simulink model "Dual_Parallel_IPMSM_Rotate_HFI"  (R2022b)
settings: Solver=FixedStepAuto  StartTime=0.0  StopTime=20  FixedStep=1e-7  RelTol=1e-3
undefined symbols (not defined in the file): DiscIntNeverNeededParam
libraries: dsparch4 x6, slpidlib x4, spsSecondOrderFilterLib x2, spsPermanentMagnetSynchronousMachineLib x2, spsDCVoltageSourceLib x1, simulink x1, spsUniversalBridgeLib x1, spspowerguiLib x1
settings Model: Creator=SSC  LastModifiedBy=SSC

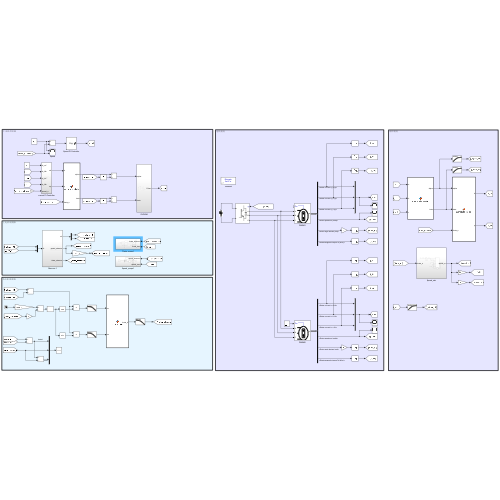
[thumbnail: Simulink's stored preview of the top-level diagram]
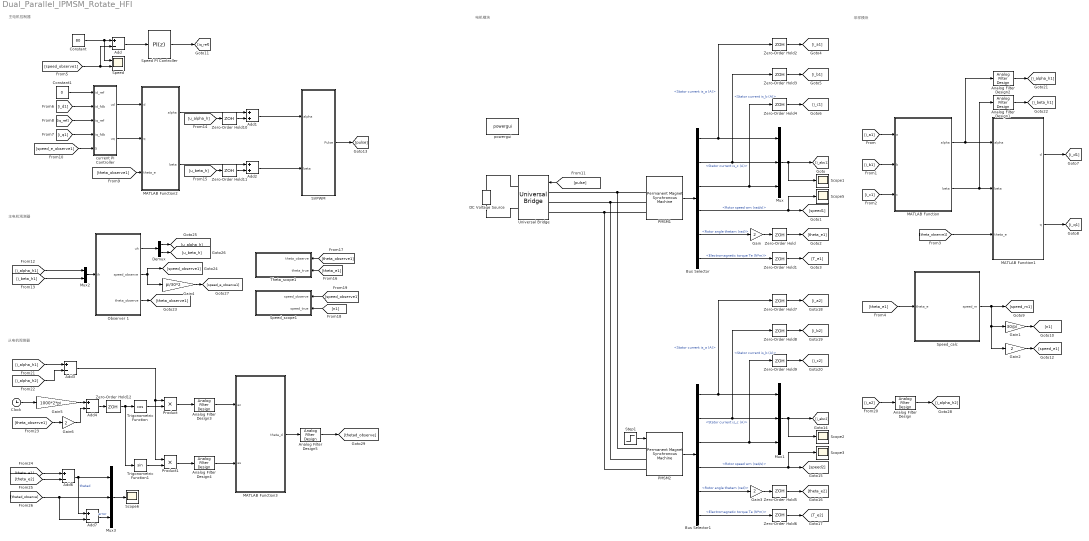
== system Dual_Parallel_IPMSM_Rotate_HFI ==
  note: 主电机观测器
  note: 采样模块
  note: 电机模块
  note: 主电机控制器
  note: 从电机观测器
  Add{,3..4,6..7} (5 alike) : Sum  Inputs=+-
  Add1 : Sum
  Add2 : Sum
  Analog Filter Design : dsparch4/Analog Filter Design  method=Butterworth  filttype=Highpass  N=1  Wlo=200*2*pi  Whi=80  Rp=2  Rs=40
  Analog Filter Design1 : dsparch4/Analog Filter Design  method=Butterworth  filttype=Highpass  N=1  Wlo=200*2*pi  Whi=80  Rp=2  Rs=40
  Analog Filter Design2 : dsparch4/Analog Filter Design  method=Butterworth  filttype=Highpass  N=1  Wlo=200*2*pi  Whi=80  Rp=2  Rs=40
  Analog Filter Design3 : dsparch4/Analog Filter Design  method=Butterworth  filttype=Lowpass  N=1  Wlo=2*2*pi  Whi=80  Rp=2  Rs=40
  Analog Filter Design4 : dsparch4/Analog Filter Design  method=Butterworth  filttype=Lowpass  N=1  Wlo=2*2*pi  Whi=80  Rp=2  Rs=40
  Analog Filter Design5 : dsparch4/Analog Filter Design  method=Butterworth  filttype=Lowpass  N=1  Wlo=1*2*pi  Whi=80  Rp=2  Rs=40
  Bus Selector : BusSelector  OutputSignals=Stator current is_a (A),Stator current is_b (A),Stator current is_c (A),Rotor speed wm (rad/s),Rotor angle thetam (rad),Electromagnetic torque Te (N*m)
  Bus Selector1 : BusSelector  OutputSignals=Stator current is_a (A),Stator current is_b (A),Stator current is_c (A),Rotor speed wm (rad/s),Rotor angle thetam (rad),Electromagnetic torque Te (N*m)
  Clock : Clock
  Constant : Constant  Value=80
  Constant1 : Constant  Value=0
  DC Voltage Source : spsDCVoltageSourceLib/DC Voltage Source  Amplitude=600  Measurements=None
  Demux : Demux  Outputs=2
  Gain{,2..3,6} (4 alike) : Gain  Gain=2
  Gain1 : Gain  Gain=30/pi
  Gain4 : Gain  Gain=pi/30*2
  Gain5 : Gain  Gain=1000*2*pi
  MATLAB Function : MATLAB Function  TreatAsAtomicUnit=on
  MATLAB Function1 : MATLAB Function  TreatAsAtomicUnit=on
  MATLAB Function2 : MATLAB Function  TreatAsAtomicUnit=on
  MATLAB Function3 : MATLAB Function  TreatAsAtomicUnit=on
  Mux : Mux  Inputs=3
  Mux1 : Mux  Inputs=3
  Mux2 : Mux  Inputs=2
  Mux3 : Mux  Inputs=3
  Observer 1 : Subsystem
  PMSM1 : spsPermanentMagnetSynchronousMachineLib/Permanent Magnet Synchronous Machine  NbPhases=3  FluxDistribution=Sinusoidal  RotorType=Salient-pole  MechanicalLoad=Torque Tm  PresetModel=No  ShowDetailedParameters=on  MeasurementBus=off  Resistance=0.91  Inductance=8.5e-3  dqInductances=[0.00396,0.00796]  La=8.5e-3  MachineConstant=Flux linkage established by magnets (V.s)  Flux=0.446  VoltageCst=161.7909  TorqueCst=1.338  Flat=120  Mechanical=[0.074 0.008 2 0]  PolePairs=4  InitialConditions=[0, 0, 0 ,0]  InitialConditions5ph=[0 0 0 0 0 0]  RefAngle=Aligned with phase A axis (original Park)  IterativeDiscreteModel=Trapezoidal non iterative  TsBlock=-1  TsPowergui=0
  PMSM2 : spsPermanentMagnetSynchronousMachineLib/Permanent Magnet Synchronous Machine  NbPhases=3  FluxDistribution=Sinusoidal  RotorType=Salient-pole  MechanicalLoad=Torque Tm  PresetModel=No  ShowDetailedParameters=on  MeasurementBus=off  Resistance=0.91  Inductance=8.5e-3  dqInductances=[0.00396,0.00796]  La=8.5e-3  MachineConstant=Flux linkage established by magnets (V.s)  Flux=0.446  VoltageCst=161.7909  TorqueCst=1.338  Flat=120  Mechanical=[0.074 0.008 2 0]  PolePairs=4  InitialConditions=[0, 0, 0 ,0]  InitialConditions5ph=[0 0 0 0 0 0]  RefAngle=Aligned with phase A axis (original Park)  IterativeDiscreteModel=Trapezoidal non iterative  TsBlock=-1  TsPowergui=0
  Product : Product
  Product1 : Product
  SVPWM : Subsystem
  Scope{1..3,5..6} (5 alike) : Scope
  Speed : Scope  NumInputPorts=2
  Speed PI Controller : slpidlib/PID Controller  Controller=PI  Form=Parallel  TimeDomain=Discrete-time  UseExternalTs=off  SampleTime=1e-4  IntegratorMethod=Forward Euler  FilterMethod=Forward Euler  ControllerParametersSource=internal  P=3.736/60  I=44.84/60  UseKiTs=off  D=0  N=100  UseFilter=on  TunerSelectOption=Transfer Function Based (PID Tuner App)  InitialConditionSource=internal  InitialConditionForIntegrator=0  InitialConditionForFilter=0  DifferentiatorICPrevScaledInput=0  ExternalReset=none  TrackingMode=off  Kt=1  LimitOutput=on  SatLimitsSource=internal  UpperSaturationLimit=20  LowerSaturationLimit=-20  LinearizeAsGain=on  AntiWindupMode=clamping  Kb=1  LimitIntegrator=off  UpperIntegratorSaturationLimit=5.65  LowerIntegratorSaturationLimit=-inf  POutMin=[]  POutMax=[]  IOutMin=[]  IOutMax=[]  DOutMin=[]  DOutMax=[]  NOutMin=[]  NOutMax=[]  SumOutMin=[]  SumOutMax=[]  SaturationOutMin=[]  SaturationOutMax=[]  PParamMin=[]  PParamMax=[]  IParamMin=[]  IParamMax=[]  DParamMin=[]  DParamMax=[]  NParamMin=[]  NParamMax=[]  KbParamMin=[]  KbParamMax=[]  KtParamMin=[]  KtParamMax=[]  KbOutMin=[]  KbOutMax=[]  KtOutMin=[]  KtOutMax=[]  IntegratorOutMin=[]  IntegratorOutMax=[]  FilterOutMin=[]  FilterOutMax=[]  SumI1OutMin=[]  SumI1OutMax=[]  SumI2OutMin=[]  SumI2OutMax=[]  SumI3OutMin=[]  SumI3OutMax=[]  SumI4OutMin=[]  SumI4OutMax=[]  SumDOutMin=[]  SumDOutMax=[]  DifferentiatorOutMin=[]  DifferentiatorOutMax=[]  FilterDiffOutCoefMin=[]  FilterDiffOutCoefMax=[]  ReciprocalOutMin=[]  ReciprocalOutMax=[]  SumDenOutMin=[]  SumDenOutMax=[]  SumNumOutMin=[]  SumNumOutMax=[]  DivideOutMin=[]  DivideOutMax=[]  UdiffTsProdOutMin=[]  UdiffTsProdOutMax=[]  NTsProdOutMin=[]  NTsProdOutMax=[]  UintegralTsProdOutMin=[]  UintegralTsProdOutMax=[]  UngainTsProdOutMin=[]  UngainTsProdOutMax=[]  ClampingZeroOutDataTypeStr=Inherit: Inherit via back propagation  ClampingZeroOutMin=[]  ClampingZeroOutMax=[]  FilterDenConstantOutDataTypeStr=Inherit: Inherit via back propagation  FilterDenConstantOutMin=[]  FilterDenConstantOutMax=[]  PCopyOutDataTypeStr=Inherit: Inherit via back propagation  PCopyOutMin=[]  PCopyOutMax=[]  NCopyOutDataTypeStr=Inherit: Inherit via back propagation  NCopyOutMin=[]  NCopyOutMax=[]  IntegratorContinuousStateAttributes=''  IntegratorStateMustResolveToSignalObject=off  IntegratorRTWStateStorageClass=Auto  FilterContinuousStateAttributes=''  FilterStateMustResolveToSignalObject=off  FilterRTWStateStorageClass=Auto  ParallelPVariant=InternalParameters  IdealPVariant=Disabled  IVariant=InternalParameters  DVariant=Disabled  IntegratorVariant=Discrete  SatVariant=Enabled  AWVariant=DiscClampingParallel  PCopyVariant=Disabled  TRVariant=Disabled  FdbkBlocksVariant=Forward  IdealPFdbkVariant=Disabled  SatFdbkVariant=Disabled  DerivativeFilterVariant=Disabled  NVariant=Disabled  NCopyVariant=Disabled_SignalSpec  FilterICVariant=Disabled  IntegratorICVariant=InternalICs  ExternalResetVariant=Disabled  TRSumVariant=Passthrough  SumFdbkVariant=Disabled  SumVariant=Sum_PI  TsampFilterVariant=InternalTs  TsampNgainVariant=Passthrough  TsampIntegralVariant=Passthrough  ExternalSaturationOutDataTypeStr=Inherit: Same as second input
  Speed_calc : Subsystem
  Speed_scope1 : Subsystem
  Step1 : Step  After=0.01  SampleTime=0
  Theta_scope1 : Subsystem
  Trigonometric Function : Trigonometry  Operator=cos
  Trigonometric Function1 : Trigonometry
  Universal Bridge : spsUniversalBridgeLib/Universal Bridge  Arms=3  SnubberResistance=1e5  SnubberCapacitance=inf  Device=IGBT / Diodes  Ron=1e-3  Lon=0  ForwardVoltages="[  0  0  ]"  ForwardVoltage=0  GTOparameters=[ 10e-6 , 20e-6 ]  IGBTparameters=[ 1e-6 , 2e-6 ]  Measurements=None  Measurements_2=None  converterType=Rectifier
  Zero-Order Hold{,1..12} (13 alike) : ZeroOrderHold  SampleTime=1e-4
  current PI Controller : Subsystem
  powergui : spspowerguiLib/powergui  Priority=1  SimulationMode=Discrete  SampleTime=5e-7  frequency=60  Iterations=50  frequencyindice=0  Pbase=100e6  ErrMax=1e-4  UnitsV=kV  UnitsW=MW  buscounter=0  FunctionMessages=off  echomessages=off  EnableUseOfTLC=off  CurrentSourceSwitches=off  DisableSnubberDevices=off  DisableRonSwitches=off  DisableVfSwitches=off  DisplayEquations=off  AutomaticDiscreteSolvers=off  SolverType=Tustin/Backward Euler (TBE)  Interpol=off  ExternalGateDelay=off  methode=off  Ts=100  x0status=blocks  SPID=on  SwTol=0  HookPort=off  NonlinearTolerance=1e-4  nMaxIteration=100  ContinueOnMaxIteration=off  RestoreLinks=warning  ResistiveCurrentMeasurement=off  Frange=[0:2:500]  Ylog=off  Xlog=on  ShowGrid=off  save=off  variable=ZData  structure=0  ZoomFFT=off  StartTime=0.0  cycles=1  DisplayStyle=1  fundamental=60  FreqAxis=off  MaxFrequency=1000  frequencyindicesteady=1  RmsSteady=1  display=off
  wires:
  Zero-Order Hold4/1 -> [i_c1]
  current PI Controller/2(uq) -> MATLAB Function2/2(q)
  Constant1/1 -> current PI Controller/1(id_ref)
  [theta_observe1] -> MATLAB Function1/3(theta_e)
  SVPWM/1(Pulse) -> [pulse]
  current PI Controller/1(ud) -> MATLAB Function2/1(d)
  Speed PI Controller/1 -> [iq_ref]
  [theta_observe1] -> MATLAB Function2/3(theta_e)
  [iq_ref] -> current PI Controller/3(iq_ref)
  [speed_e_observe1] -> current PI Controller/5(speed_e)
  Speed_calc/1(speed_m) -> Gain2/1, Gain1/1, [speed_m1]
  Constant/1 -> Speed/1, Add/1
  Bus Selector/6 -> Zero-Order Hold1/1  "<Electromagnetic torque Te (N*m)>"
  Gain2/1 -> [speed_e1]
  PMSM1/1 -> Bus Selector/1
  MATLAB Function1/1(d) -> [i_d1]
  Add/1 -> Speed PI Controller/1
  [i_b1] -> MATLAB Function/2(b)
  [i_c1] -> MATLAB Function/3(c)
  Gain1/1 -> [n1]
  MATLAB Function1/2(q) -> [i_q1]
  [pulse] -> Universal Bridge/1
  Zero-Order Hold1/1 -> [T_e1]
  Bus Selector/1 -> Zero-Order Hold2/1, Mux/1  "<Stator current is_a (A)>"
  Bus Selector/5 -> Gain/1  "<Rotor angle thetam (rad)>"
  Bus Selector/2 -> Zero-Order Hold3/1, Mux/2  "<Stator current is_b (A)>"
  Mux/1 -> Scope1/1, [i_abc1]
  Gain/1 -> Zero-Order Hold/1
  Bus Selector/3 -> Zero-Order Hold4/1, Mux/3  "<Stator current is_c (A)>"
  [speed_observe1] -> Add/2, Speed/2
  Zero-Order Hold2/1 -> [i_a1]
  Zero-Order Hold/1 -> [theta_e1]
  [i_d1] -> current PI Controller/2(id_fdb)
  MATLAB Function/2(beta) -> Analog Filter Design1/1, MATLAB Function1/2(beta)
  [theta_e1] -> Speed_calc/1(theta_e)
  Zero-Order Hold3/1 -> [i_b1]
  [i_a1] -> MATLAB Function/1(a)
  Bus Selector/4 -> Scope5/1, [speed1]  "<Rotor speed wm (rad/s)>"
  MATLAB Function/1(alpha) -> Analog Filter Design2/1, MATLAB Function1/1(alpha)
  [i_q1] -> current PI Controller/4(iq_fdb)
  Zero-Order Hold5/1 -> [theta_e2]
  Zero-Order Hold8/1 -> [i_b2]
  Bus Selector1/3 -> Zero-Order Hold9/1, Mux1/3  "<Stator current is_c (A)>"
  Zero-Order Hold7/1 -> [i_a2]
  Bus Selector1/1 -> Zero-Order Hold7/1, Mux1/1  "<Stator current is_a (A)>"
  Bus Selector1/4 -> Scope3/1, [speed2]  "<Rotor speed wm (rad/s)>"
  Bus Selector1/6 -> Zero-Order Hold6/1  "<Electromagnetic torque Te (N*m)>"
  Gain3/1 -> Zero-Order Hold5/1
  Bus Selector1/2 -> Zero-Order Hold8/1, Mux1/2  "<Stator current is_b (A)>"
  Zero-Order Hold6/1 -> [T_e2]
  Mux1/1 -> Scope2/1, [i_abc2]
  PMSM2/1 -> Bus Selector1/1
  Zero-Order Hold9/1 -> [i_c2]
  Bus Selector1/5 -> Gain3/1  "<Rotor angle thetam (rad)>"
  MATLAB Function2/1(alpha) -> Add1/1
  MATLAB Function2/2(beta) -> Add2/1
  Zero-Order Hold10/1 -> Add1/2
  Zero-Order Hold11/1 -> Add2/2
  Analog Filter Design1/1 -> [i_beta_h1]
  Analog Filter Design2/1 -> [i_alpha_h1]
  Observer 1/1(uh) -> Demux/1
  Mux2/1 -> Observer 1/1(ih)
  [i_alpha_h1] -> Mux2/1
  [i_beta_h1] -> Mux2/2
  Observer 1/3(theta_observe) -> [theta_observe1]
  Observer 1/2(speed_observe) -> [speed_observe1], Gain4/1
  [u_alpha_h] -> Zero-Order Hold10/1
  [u_beta_h] -> Zero-Order Hold11/1
  Demux/2 -> [u_beta_h]
  Demux/1 -> [u_alpha_h]
  [theta_observe1] -> Theta_scope1/1(theta_observe)
  [theta_e1] -> Theta_scope1/2(theta_true)
  [n1] -> Speed_scope1/2(speed_true)
  [speed_observe1] -> Speed_scope1/1(speed_observe)
  Gain4/1 -> [speed_e_observe1]
  Analog Filter Design/1 -> [i_alpha_h2]
  [i_a2] -> Analog Filter Design/1
  [i_alpha_h1] -> Add3/1
  [i_alpha_h2] -> Add3/2
  Clock/1 -> Gain5/1
  Gain5/1 -> Add4/1
  [theta_observe1] -> Gain6/1
  Add3/1 -> Product1/1, Product/1
  Product/1 -> Analog Filter Design3/1
  Trigonometric Function1/1 -> Product1/2
  Product1/1 -> Analog Filter Design4/1
  Analog Filter Design3/1 -> MATLAB Function3/1(ec)
  Analog Filter Design4/1 -> MATLAB Function3/2(es)
  [theta_e1] -> Add6/1
  [theta_e2] -> Add6/2
  Add6/1 -> Mux3/1, Add7/1  "thetad"
  [thetad_observe] -> Add7/2, Mux3/2
  Mux3/1 -> Scope6/1
  Add7/1 -> Mux3/3  "error"
  Add1/1 -> SVPWM/1(alpha)
  Add2/1 -> SVPWM/2(beta)
  Gain6/1 -> Add4/2
  Trigonometric Function/1 -> Product/2
  Add4/1 -> Zero-Order Hold12/1
  Zero-Order Hold12/1 -> Trigonometric Function1/1, Trigonometric Function/1
  MATLAB Function3/1(theta_d) -> Analog Filter Design5/1
  Analog Filter Design5/1 -> [thetad_observe]
  Step1/1 -> PMSM2/1
  connections:
  Universal Bridge/RConn1 -- DC Voltage Source/RConn1
  PMSM1/LConn2 -- PMSM2/LConn2 -- Universal Bridge/LConn2
  DC Voltage Source/LConn1 -- Universal Bridge/RConn2
  PMSM1/LConn1 -- PMSM2/LConn1 -- Universal Bridge/LConn1
  PMSM1/LConn3 -- PMSM2/LConn3 -- Universal Bridge/LConn3

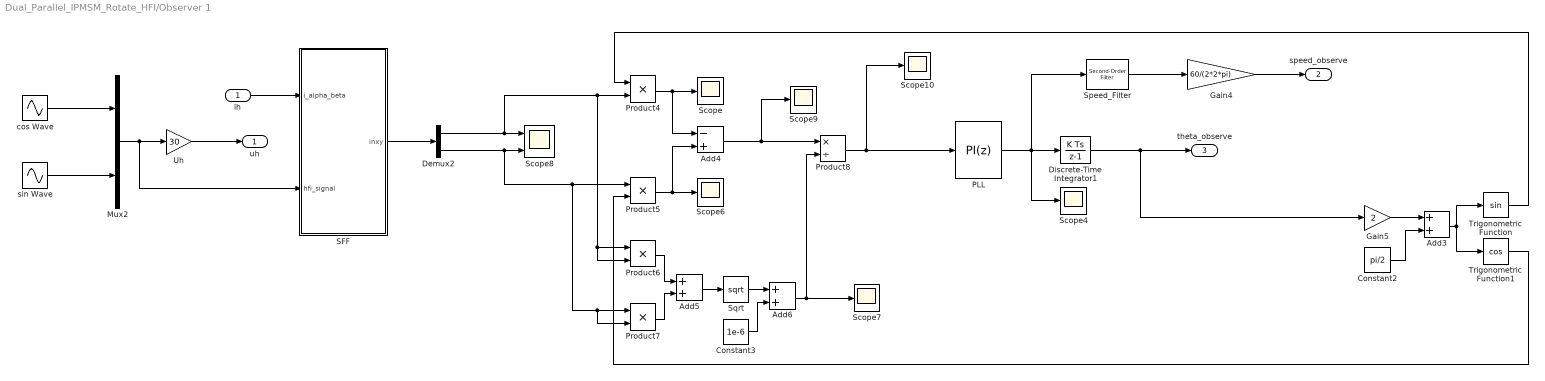
== system Dual_Parallel_IPMSM_Rotate_HFI/Observer 1 ==
  ih : Inport
  Add3 : Sum
  Add4 : Sum  Inputs=-+
  Add5 : Sum
  Add6 : Sum
  Constant2 : Constant  Value=pi/2  SampleTime=-1
  Constant3 : Constant  Value=1e-6  SampleTime=-1
  Demux2 : Demux  Outputs=2
  Discrete-Time Integrator1 : DiscreteIntegrator  SampleTime=-1  ICPrevOutput=DiscIntNeverNeededParam  ICPrevScaledInput=DiscIntNeverNeededParam
  Gain4 : Gain  Gain=60/(2*2*pi)
  Gain5 : Gain  Gain=2
  Mux2 : Mux  Inputs=2
  PLL : slpidlib/PID Controller  Controller=PI  Form=Parallel  TimeDomain=Discrete-time  UseExternalTs=off  SampleTime=1e-4  IntegratorMethod=Forward Euler  FilterMethod=Forward Euler  ControllerParametersSource=internal  P=500  I=4000  UseKiTs=off  D=0  N=100  UseFilter=on  TunerSelectOption=Transfer Function Based (PID Tuner App)  InitialConditionSource=internal  InitialConditionForIntegrator=0  InitialConditionForFilter=0  DifferentiatorICPrevScaledInput=0  ExternalReset=none  TrackingMode=off  Kt=1  LimitOutput=on  SatLimitsSource=internal  UpperSaturationLimit=100*2*pi  LowerSaturationLimit=-100*2*pi  LinearizeAsGain=on  AntiWindupMode=clamping  Kb=1  LimitIntegrator=off  UpperIntegratorSaturationLimit=inf  LowerIntegratorSaturationLimit=-inf  POutMin=[]  POutMax=[]  IOutMin=[]  IOutMax=[]  DOutMin=[]  DOutMax=[]  NOutMin=[]  NOutMax=[]  SumOutMin=[]  SumOutMax=[]  SaturationOutMin=[]  SaturationOutMax=[]  PParamMin=[]  PParamMax=[]  IParamMin=[]  IParamMax=[]  DParamMin=[]  DParamMax=[]  NParamMin=[]  NParamMax=[]  KbParamMin=[]  KbParamMax=[]  KtParamMin=[]  KtParamMax=[]  KbOutMin=[]  KbOutMax=[]  KtOutMin=[]  KtOutMax=[]  IntegratorOutMin=[]  IntegratorOutMax=[]  FilterOutMin=[]  FilterOutMax=[]  SumI1OutMin=[]  SumI1OutMax=[]  SumI2OutMin=[]  SumI2OutMax=[]  SumI3OutMin=[]  SumI3OutMax=[]  SumI4OutMin=[]  SumI4OutMax=[]  SumDOutMin=[]  SumDOutMax=[]  DifferentiatorOutMin=[]  DifferentiatorOutMax=[]  FilterDiffOutCoefMin=[]  FilterDiffOutCoefMax=[]  ReciprocalOutMin=[]  ReciprocalOutMax=[]  SumDenOutMin=[]  SumDenOutMax=[]  SumNumOutMin=[]  SumNumOutMax=[]  DivideOutMin=[]  DivideOutMax=[]  UdiffTsProdOutMin=[]  UdiffTsProdOutMax=[]  NTsProdOutMin=[]  NTsProdOutMax=[]  UintegralTsProdOutMin=[]  UintegralTsProdOutMax=[]  UngainTsProdOutMin=[]  UngainTsProdOutMax=[]  ClampingZeroOutDataTypeStr=Inherit: Inherit via back propagation  ClampingZeroOutMin=[]  ClampingZeroOutMax=[]  FilterDenConstantOutDataTypeStr=Inherit: Inherit via back propagation  FilterDenConstantOutMin=[]  FilterDenConstantOutMax=[]  PCopyOutDataTypeStr=Inherit: Inherit via back propagation  PCopyOutMin=[]  PCopyOutMax=[]  NCopyOutDataTypeStr=Inherit: Inherit via back propagation  NCopyOutMin=[]  NCopyOutMax=[]  IntegratorContinuousStateAttributes=''  IntegratorStateMustResolveToSignalObject=off  IntegratorRTWStateStorageClass=Auto  FilterContinuousStateAttributes=''  FilterStateMustResolveToSignalObject=off  FilterRTWStateStorageClass=Auto  ParallelPVariant=InternalParameters  IdealPVariant=Disabled  IVariant=InternalParameters  DVariant=Disabled  IntegratorVariant=Discrete  SatVariant=Enabled  AWVariant=DiscClampingParallel  PCopyVariant=Disabled  TRVariant=Disabled  FdbkBlocksVariant=Forward  IdealPFdbkVariant=Disabled  SatFdbkVariant=Disabled  DerivativeFilterVariant=Disabled  NVariant=Disabled  NCopyVariant=Disabled_SignalSpec  FilterICVariant=Disabled  IntegratorICVariant=InternalICs  ExternalResetVariant=Disabled  TRSumVariant=Passthrough  SumFdbkVariant=Disabled  SumVariant=Sum_PI  TsampFilterVariant=InternalTs  TsampNgainVariant=Passthrough  TsampIntegralVariant=Passthrough  ExternalSaturationOutDataTypeStr=Inherit: Same as second input
  Product{4..7} (4 alike) : Product
  Product8 : Product  Inputs=*/
  SFF : Subsystem
  Scope{,4,6..7,9..10} (6 alike) : Scope
  Scope8 : Scope  NumInputPorts=2
  Speed_Filter : spsSecondOrderFilterLib/Second-Order Filter  FilterType=Lowpass  Fo=500  Zeta=0.3  Ts=1e-4  Initialize=off  Vac_Init="[0,  0,  60]"  Vdc_Init=0  PlotResponse=off  FreqRange=[0, 500, 1]
      settings: LibrarySourceBlock=|
      | sps_lib/Control/Filters/Second-Order
      | Filter
  Sqrt : Sqrt
  Trigonometric Function : Trigonometry
  Trigonometric Function1 : Trigonometry  Operator=cos
  Uh : Gain  Gain=30
  cos Wave : Sin  Frequency=1000*2*pi  Phase=pi/2
  sin Wave : Sin  Frequency=1000*2*pi
  uh : Outport
  speed_observe : Outport  Port=2  VectorParamsAs1DForOutWhenUnconnected=off
  theta_observe : Outport  Port=3  VectorParamsAs1DForOutWhenUnconnected=off
  wires:
  Constant3/1 -> Add6/2
  ih/1 -> SFF/1(i_alpha_beta)
  Product4/1 -> Add4/1, Scope/1
  Constant2/1 -> Add3/2
  SFF/1(inxy) -> Demux2/1
  Product8/1 -> PLL/1, Scope10/1
  Sqrt/1 -> Add6/1
  Add6/1 -> Product8/2, Scope7/1
  Demux2/1 -> Product6/2, Product6/1, Product4/2, Scope8/1
  PLL/1 -> Scope4/1, Speed_Filter/1, Discrete-Time Integrator1/1
  Product5/1 -> Scope6/1, Add4/2
  cos Wave/1 -> Mux2/1
  Product7/1 -> Add5/2
  Uh/1 -> uh/1
  Add3/1 -> Trigonometric Function/1, Trigonometric Function1/1
  Add5/1 -> Sqrt/1
  Product6/1 -> Add5/1
  Gain4/1 -> speed_observe/1
  Mux2/1 -> SFF/2(hfi_signal), Uh/1
  Add4/1 -> Scope9/1, Product8/1
  Trigonometric Function/1 -> Product4/1
  Speed_Filter/1 -> Gain4/1
  Gain5/1 -> Add3/1
  Discrete-Time Integrator1/1 -> theta_observe/1, Gain5/1
  Demux2/2 -> Product7/2, Product7/1, Product5/1, Scope8/2
  sin Wave/1 -> Mux2/2
  Trigonometric Function1/1 -> Product5/2

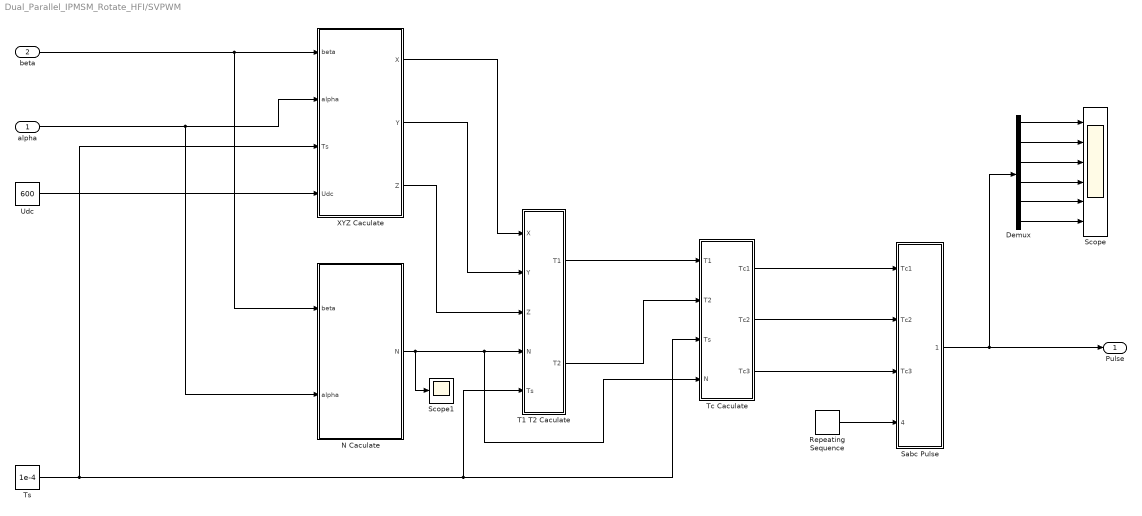
== system Dual_Parallel_IPMSM_Rotate_HFI/SVPWM ==
  alpha : Inport
  beta : Inport  Port=2
  Demux : Demux  Outputs=6
  N Caculate : Subsystem
  Repeating Sequence : simulink/Sources/Repeating Sequence  rep_seq_t=[0 0.5*1e-4 1e-4]  rep_seq_y=[0 0.5*1e-4 0]
  Sabc Pulse : Subsystem
  Scope : Scope  NumInputPorts=6
  Scope1 : Scope
  T1 T2 Caculate : Subsystem
  Tc Caculate : Subsystem
  Ts : Constant  Value=1e-4
  "Udc " : Constant  Value=600
  XYZ Caculate : Subsystem
  Pulse : Outport  VectorParamsAs1DForOutWhenUnconnected=off
  wires:
  beta/1 -> N Caculate/1(beta), XYZ Caculate/1(beta)
  alpha/1 -> N Caculate/2(alpha), XYZ Caculate/2(alpha)
  XYZ Caculate/1(X) -> T1 T2 Caculate/1(X)
  XYZ Caculate/2(Y) -> T1 T2 Caculate/2(Y)
  XYZ Caculate/3(Z) -> T1 T2 Caculate/3(Z)
  N Caculate/1(N) -> Scope1/1, Tc Caculate/4(N), T1 T2 Caculate/4(N)
  Ts/1 -> XYZ Caculate/3("Ts "), Tc Caculate/3(Ts), T1 T2 Caculate/5("Ts ")
  T1 T2 Caculate/1(T1) -> Tc Caculate/1(T1)
  T1 T2 Caculate/2(T2) -> Tc Caculate/2(T2)
  Tc Caculate/1(Tc1) -> Sabc Pulse/1(Tc1)
  Tc Caculate/2(Tc2) -> Sabc Pulse/2(Tc2)
  Tc Caculate/3(Tc3) -> Sabc Pulse/3(Tc3)
  Sabc Pulse/1("Pulse ") -> Demux/1, Pulse/1
  "Udc "/1 -> XYZ Caculate/4(Udc)
  Repeating Sequence/1 -> Sabc Pulse/4(Wave)
  Demux/1 -> Scope/1
  Demux/2 -> Scope/2
  Demux/3 -> Scope/3
  Demux/4 -> Scope/4
  Demux/5 -> Scope/5
  Demux/6 -> Scope/6

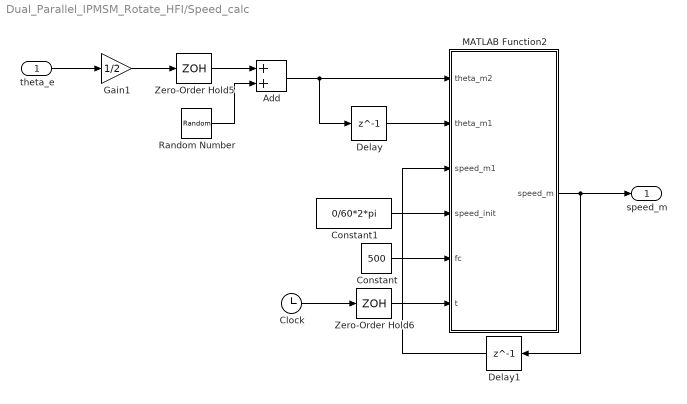
== system Dual_Parallel_IPMSM_Rotate_HFI/Speed_calc ==
  theta_e : Inport
  Add : Sum
  Clock : Clock
  Constant : Constant  Value=500
  Constant1 : Constant  Value=0/60*2*pi
  Delay : Delay  DelayLength=1  InitialCondition=0
  Delay1 : Delay  DelayLength=1  InitialCondition=0
  Gain1 : Gain  Gain=1/2
  MATLAB Function2 : MATLAB Function  TreatAsAtomicUnit=on
  Random Number : RandomNumber  Mean=1.25e-9  Variance=1.25e-9  SampleTime=1e-4
  Zero-Order Hold5 : ZeroOrderHold  SampleTime=1e-4
  Zero-Order Hold6 : ZeroOrderHold  SampleTime=1e-4
  speed_m : Outport
  wires:
  Delay/1 -> MATLAB Function2/2(theta_m1)
  Constant1/1 -> MATLAB Function2/4(speed_init)
  Clock/1 -> Zero-Order Hold6/1
  Add/1 -> Delay/1, MATLAB Function2/1(theta_m2)
  Constant/1 -> MATLAB Function2/5(fc)
  Delay1/1 -> MATLAB Function2/3(speed_m1)
  MATLAB Function2/1(speed_m) -> speed_m/1, Delay1/1
  theta_e/1 -> Gain1/1
  Zero-Order Hold6/1 -> MATLAB Function2/6(t)
  Zero-Order Hold5/1 -> Add/1
  Gain1/1 -> Zero-Order Hold5/1
  Random Number/1 -> Add/2

== system Dual_Parallel_IPMSM_Rotate_HFI/Speed_scope1 ==
  speed_observe : Inport
  speed_true : Inport  Port=2
  Add : Sum  Inputs=+-
  Mux : Mux  Inputs=3
  speed : Scope
  wires:
  Mux/1 -> speed/1
  speed_true/1 -> Mux/2, Add/1
  speed_observe/1 -> Mux/1, Add/2
  Add/1 -> Mux/3  "speed_error"

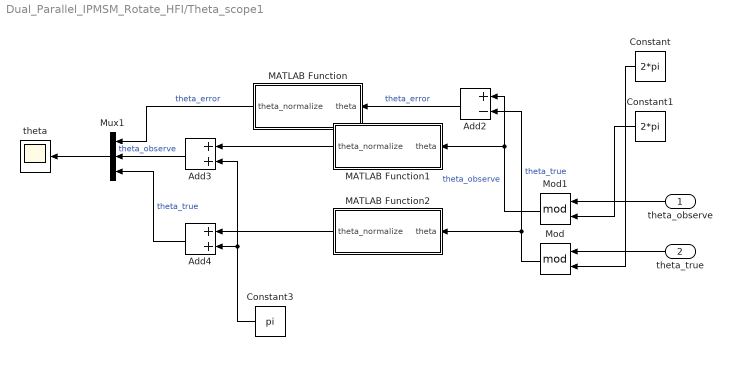
== system Dual_Parallel_IPMSM_Rotate_HFI/Theta_scope1 ==
  theta_observe : Inport
  theta_true : Inport  Port=2
  Add2 : Sum  Inputs=+-
  Add3 : Sum
  Add4 : Sum
  Constant : Constant  Value=2*pi
  Constant1 : Constant  Value=2*pi
  Constant3 : Constant  Value=pi
  MATLAB Function : MATLAB Function  TreatAsAtomicUnit=on
  MATLAB Function1 : MATLAB Function  TreatAsAtomicUnit=on
  MATLAB Function2 : MATLAB Function  TreatAsAtomicUnit=on
  Mod : Math  Operator=mod  SignedPower=on
  Mod1 : Math  Operator=mod  SignedPower=on
  Mux1 : Mux  Inputs=3
  theta : Scope
  wires:
  Add4/1 -> Mux1/3  "theta_true"
  Constant1/1 -> Mod1/2
  Constant/1 -> Mod/2
  MATLAB Function2/1(theta_normalize) -> Add4/1
  Mod/1 -> Add2/2, MATLAB Function2/1(theta)  "theta_true"
  Mux1/1 -> theta/1
  theta_observe/1 -> Mod1/1
  Constant3/1 -> Add4/2, Add3/2
  MATLAB Function/1(theta_normalize) -> Mux1/1  "theta_error"
  MATLAB Function1/1(theta_normalize) -> Add3/1
  Mod1/1 -> Add2/1, MATLAB Function1/1(theta)  "theta_observe"
  Add3/1 -> Mux1/2  "theta_observe"
  Add2/1 -> MATLAB Function/1(theta)  "theta_error"
  theta_true/1 -> Mod/1

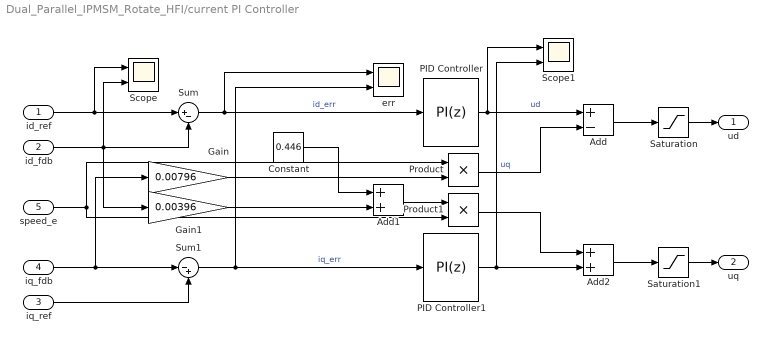
== system Dual_Parallel_IPMSM_Rotate_HFI/current PI Controller ==
  id_ref : Inport
  id_fdb : Inport  Port=2
  iq_ref : Inport  Port=3
  iq_fdb : Inport  Port=4
  speed_e : Inport  Port=5
  Add : Sum  Inputs=+-
  Add1 : Sum
  Add2 : Sum
  Constant : Constant  Value=0.446
  Gain : Gain  Gain=0.00796
  Gain1 : Gain  Gain=0.00396
  PID Controller : slpidlib/PID Controller  Controller=PI  Form=Parallel  TimeDomain=Discrete-time  UseExternalTs=off  SampleTime=1e-4  IntegratorMethod=Forward Euler  FilterMethod=Forward Euler  ControllerParametersSource=internal  P=0.00396 * 400  I=0.91 * 400  UseKiTs=off  D=0  N=100  UseFilter=on  TunerSelectOption=Transfer Function Based (PID Tuner App)  InitialConditionSource=internal  InitialConditionForIntegrator=0  InitialConditionForFilter=0  DifferentiatorICPrevScaledInput=0  ExternalReset=none  TrackingMode=off  Kt=1  LimitOutput=on  SatLimitsSource=internal  UpperSaturationLimit=600/sqrt(3)  LowerSaturationLimit=-600/sqrt(3)  LinearizeAsGain=on  AntiWindupMode=clamping  Kb=1  LimitIntegrator=off  UpperIntegratorSaturationLimit=inf  LowerIntegratorSaturationLimit=-inf  POutMin=[]  POutMax=[]  IOutMin=[]  IOutMax=[]  DOutMin=[]  DOutMax=[]  NOutMin=[]  NOutMax=[]  SumOutMin=[]  SumOutMax=[]  SaturationOutMin=[]  SaturationOutMax=[]  PParamMin=[]  PParamMax=[]  IParamMin=[]  IParamMax=[]  DParamMin=[]  DParamMax=[]  NParamMin=[]  NParamMax=[]  KbParamMin=[]  KbParamMax=[]  KtParamMin=[]  KtParamMax=[]  KbOutMin=[]  KbOutMax=[]  KtOutMin=[]  KtOutMax=[]  IntegratorOutMin=[]  IntegratorOutMax=[]  FilterOutMin=[]  FilterOutMax=[]  SumI1OutMin=[]  SumI1OutMax=[]  SumI2OutMin=[]  SumI2OutMax=[]  SumI3OutMin=[]  SumI3OutMax=[]  SumI4OutMin=[]  SumI4OutMax=[]  SumDOutMin=[]  SumDOutMax=[]  DifferentiatorOutMin=[]  DifferentiatorOutMax=[]  FilterDiffOutCoefMin=[]  FilterDiffOutCoefMax=[]  ReciprocalOutMin=[]  ReciprocalOutMax=[]  SumDenOutMin=[]  SumDenOutMax=[]  SumNumOutMin=[]  SumNumOutMax=[]  DivideOutMin=[]  DivideOutMax=[]  UdiffTsProdOutMin=[]  UdiffTsProdOutMax=[]  NTsProdOutMin=[]  NTsProdOutMax=[]  UintegralTsProdOutMin=[]  UintegralTsProdOutMax=[]  UngainTsProdOutMin=[]  UngainTsProdOutMax=[]  ClampingZeroOutDataTypeStr=Inherit: Inherit via back propagation  ClampingZeroOutMin=[]  ClampingZeroOutMax=[]  FilterDenConstantOutDataTypeStr=Inherit: Inherit via back propagation  FilterDenConstantOutMin=[]  FilterDenConstantOutMax=[]  PCopyOutDataTypeStr=Inherit: Inherit via back propagation  PCopyOutMin=[]  PCopyOutMax=[]  NCopyOutDataTypeStr=Inherit: Inherit via back propagation  NCopyOutMin=[]  NCopyOutMax=[]  IntegratorContinuousStateAttributes=''  IntegratorStateMustResolveToSignalObject=off  IntegratorRTWStateStorageClass=Auto  FilterContinuousStateAttributes=''  FilterStateMustResolveToSignalObject=off  FilterRTWStateStorageClass=Auto  ParallelPVariant=InternalParameters  IdealPVariant=Disabled  IVariant=InternalParameters  DVariant=Disabled  IntegratorVariant=Discrete  SatVariant=Enabled  AWVariant=DiscClampingParallel  PCopyVariant=Disabled  TRVariant=Disabled  FdbkBlocksVariant=Forward  IdealPFdbkVariant=Disabled  SatFdbkVariant=Disabled  DerivativeFilterVariant=Disabled  NVariant=Disabled  NCopyVariant=Disabled_SignalSpec  FilterICVariant=Disabled  IntegratorICVariant=InternalICs  ExternalResetVariant=Disabled  TRSumVariant=Passthrough  SumFdbkVariant=Disabled  SumVariant=Sum_PI  TsampFilterVariant=InternalTs  TsampNgainVariant=Passthrough  TsampIntegralVariant=Passthrough  ExternalSaturationOutDataTypeStr=Inherit: Same as second input
  PID Controller1 : slpidlib/PID Controller  Controller=PI  Form=Parallel  TimeDomain=Discrete-time  UseExternalTs=off  SampleTime=1e-4  IntegratorMethod=Forward Euler  FilterMethod=Forward Euler  ControllerParametersSource=internal  P=0.00796 * 400  I=0.91 * 400  UseKiTs=off  D=0  N=100  UseFilter=on  TunerSelectOption=Transfer Function Based (PID Tuner App)  InitialConditionSource=internal  InitialConditionForIntegrator=0  InitialConditionForFilter=0  DifferentiatorICPrevScaledInput=0  ExternalReset=none  TrackingMode=off  Kt=1  LimitOutput=on  SatLimitsSource=internal  UpperSaturationLimit=600/sqrt(3)  LowerSaturationLimit=-600/sqrt(3)  LinearizeAsGain=on  AntiWindupMode=clamping  Kb=1  LimitIntegrator=off  UpperIntegratorSaturationLimit=inf  LowerIntegratorSaturationLimit=-inf  POutMin=[]  POutMax=[]  IOutMin=[]  IOutMax=[]  DOutMin=[]  DOutMax=[]  NOutMin=[]  NOutMax=[]  SumOutMin=[]  SumOutMax=[]  SaturationOutMin=[]  SaturationOutMax=[]  PParamMin=[]  PParamMax=[]  IParamMin=[]  IParamMax=[]  DParamMin=[]  DParamMax=[]  NParamMin=[]  NParamMax=[]  KbParamMin=[]  KbParamMax=[]  KtParamMin=[]  KtParamMax=[]  KbOutMin=[]  KbOutMax=[]  KtOutMin=[]  KtOutMax=[]  IntegratorOutMin=[]  IntegratorOutMax=[]  FilterOutMin=[]  FilterOutMax=[]  SumI1OutMin=[]  SumI1OutMax=[]  SumI2OutMin=[]  SumI2OutMax=[]  SumI3OutMin=[]  SumI3OutMax=[]  SumI4OutMin=[]  SumI4OutMax=[]  SumDOutMin=[]  SumDOutMax=[]  DifferentiatorOutMin=[]  DifferentiatorOutMax=[]  FilterDiffOutCoefMin=[]  FilterDiffOutCoefMax=[]  ReciprocalOutMin=[]  ReciprocalOutMax=[]  SumDenOutMin=[]  SumDenOutMax=[]  SumNumOutMin=[]  SumNumOutMax=[]  DivideOutMin=[]  DivideOutMax=[]  UdiffTsProdOutMin=[]  UdiffTsProdOutMax=[]  NTsProdOutMin=[]  NTsProdOutMax=[]  UintegralTsProdOutMin=[]  UintegralTsProdOutMax=[]  UngainTsProdOutMin=[]  UngainTsProdOutMax=[]  ClampingZeroOutDataTypeStr=Inherit: Inherit via back propagation  ClampingZeroOutMin=[]  ClampingZeroOutMax=[]  FilterDenConstantOutDataTypeStr=Inherit: Inherit via back propagation  FilterDenConstantOutMin=[]  FilterDenConstantOutMax=[]  PCopyOutDataTypeStr=Inherit: Inherit via back propagation  PCopyOutMin=[]  PCopyOutMax=[]  NCopyOutDataTypeStr=Inherit: Inherit via back propagation  NCopyOutMin=[]  NCopyOutMax=[]  IntegratorContinuousStateAttributes=''  IntegratorStateMustResolveToSignalObject=off  IntegratorRTWStateStorageClass=Auto  FilterContinuousStateAttributes=''  FilterStateMustResolveToSignalObject=off  FilterRTWStateStorageClass=Auto  ParallelPVariant=InternalParameters  IdealPVariant=Disabled  IVariant=InternalParameters  DVariant=Disabled  IntegratorVariant=Discrete  SatVariant=Enabled  AWVariant=DiscClampingParallel  PCopyVariant=Disabled  TRVariant=Disabled  FdbkBlocksVariant=Forward  IdealPFdbkVariant=Disabled  SatFdbkVariant=Disabled  DerivativeFilterVariant=Disabled  NVariant=Disabled  NCopyVariant=Disabled_SignalSpec  FilterICVariant=Disabled  IntegratorICVariant=InternalICs  ExternalResetVariant=Disabled  TRSumVariant=Passthrough  SumFdbkVariant=Disabled  SumVariant=Sum_PI  TsampFilterVariant=InternalTs  TsampNgainVariant=Passthrough  TsampIntegralVariant=Passthrough  ExternalSaturationOutDataTypeStr=Inherit: Same as second input
  Product : Product
  Product1 : Product
  Saturation : Saturate  UpperLimit=600/sqrt(3)  LowerLimit=-600/sqrt(3)
  Saturation1 : Saturate  UpperLimit=600/sqrt(3)  LowerLimit=-600/sqrt(3)
  Scope : Scope  NumInputPorts=2
  Scope1 : Scope  NumInputPorts=2
  Sum : Sum  Inputs=|+-
  Sum1 : Sum  Inputs=|-+
  err : Scope  NumInputPorts=2
  ud : Outport
  uq : Outport  Port=2
  wires:
  Sum1/1 -> PID Controller1/1, err/2  "iq_err"
  id_fdb/1 -> Sum/2, Gain1/1, Scope/2
  Sum/1 -> err/1, PID Controller/1  "id_err"
  id_ref/1 -> Scope/1, Sum/1
  PID Controller1/1 -> Scope1/2, Add2/2  "uq"
  PID Controller/1 -> Add/1, Scope1/1  "ud"
  Saturation/1 -> ud/1
  Saturation1/1 -> uq/1
  iq_fdb/1 -> Sum1/1, Gain/1
  iq_ref/1 -> Sum1/2
  speed_e/1 -> Product/1, Product1/2
  Gain/1 -> Product/2
  Product/1 -> Add/2
  Add/1 -> Saturation/1
  Gain1/1 -> Add1/2
  Constant/1 -> Add1/1
  Add1/1 -> Product1/1
  Add2/1 -> Saturation1/1
  Product1/1 -> Add2/1

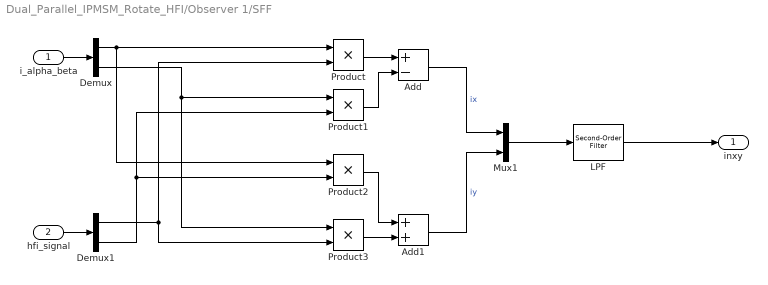
== system Dual_Parallel_IPMSM_Rotate_HFI/Observer 1/SFF ==
  i_alpha_beta : Inport
  hfi_signal : Inport  Port=2
  Add : Sum  Inputs=+-
  Add1 : Sum
  Demux : Demux  Outputs=2
  Demux1 : Demux  Outputs=2
  LPF : spsSecondOrderFilterLib/Second-Order Filter  FilterType=Lowpass  Fo=50  Zeta=0.707  Ts=1e-4  Initialize=off  Vac_Init="[0,  0,  60]"  Vdc_Init=0  PlotResponse=off  FreqRange=[0, 500, 1]
      settings: LibrarySourceBlock=|
      | sps_lib/Control/Filters/Second-Order
      | Filter
  Mux1 : Mux  Inputs=2
  Product{,1..3} (4 alike) : Product
  inxy : Outport
  wires:
  Demux/1 -> Product/1, Product2/1
  Add/1 -> Mux1/1  "ix"
  Demux1/1 -> Product3/2, Product/2
  Demux/2 -> Product1/1, Product3/1
  Mux1/1 -> LPF/1
  Demux1/2 -> Product2/2, Product1/2
  Product3/1 -> Add1/2
  Product1/1 -> Add/2
  i_alpha_beta/1 -> Demux/1
  Product/1 -> Add/1
  Product2/1 -> Add1/1
  Add1/1 -> Mux1/2  "iy"
  hfi_signal/1 -> Demux1/1
  LPF/1 -> inxy/1

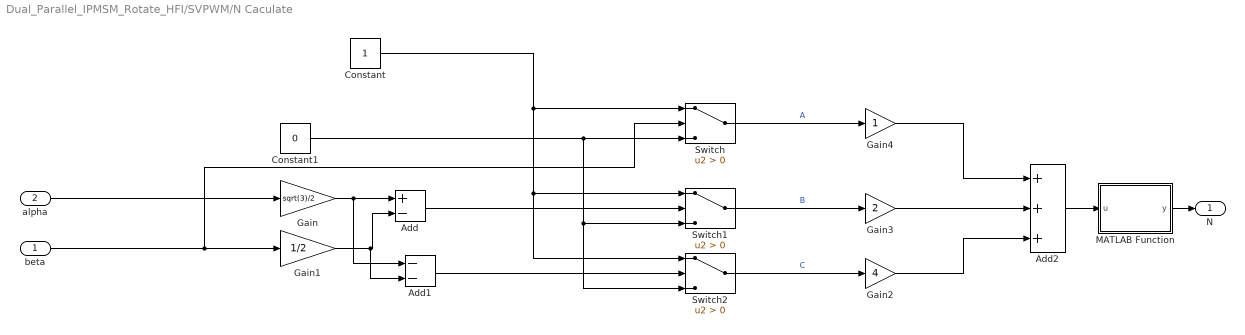
== system Dual_Parallel_IPMSM_Rotate_HFI/SVPWM/N Caculate ==
  beta : Inport
  alpha : Inport  Port=2
  Add : Sum  Inputs=+-
  Add1 : Sum  Inputs=--
  Add2 : Sum  Inputs=+++
  Constant : Constant
  Constant1 : Constant  Value=0
  Gain : Gain  Gain=sqrt(3)/2
  Gain1 : Gain  Gain=1/2
  Gain2 : Gain  Gain=4
  Gain3 : Gain  Gain=2
  Gain4 : Gain
  MATLAB Function : MATLAB Function  TreatAsAtomicUnit=on
  Switch : Switch  Criteria=u2 > Threshold  SaturateOnIntegerOverflow=off  InputSameDT=off
  Switch1 : Switch  Criteria=u2 > Threshold  SaturateOnIntegerOverflow=off  InputSameDT=off
  Switch2 : Switch  Criteria=u2 > Threshold  SaturateOnIntegerOverflow=off  InputSameDT=off
  N : Outport  VectorParamsAs1DForOutWhenUnconnected=off
  wires:
  Switch/1 -> Gain4/1  "A"
  Add/1 -> Switch1/2
  Gain/1 -> Add1/1, Add/1
  Gain3/1 -> Add2/2
  Gain2/1 -> Add2/3
  Constant/1 -> Switch/1, Switch2/1, Switch1/1
  Add1/1 -> Switch2/2
  Gain1/1 -> Add1/2, Add/2
  Add2/1 -> MATLAB Function/1(u)
  Constant1/1 -> Switch2/3, Switch1/3, Switch/3
  Gain4/1 -> Add2/1
  beta/1 -> Switch/2, Gain1/1
  Switch2/1 -> Gain2/1  "C"
  Switch1/1 -> Gain3/1  "B"
  alpha/1 -> Gain/1
  MATLAB Function/1(y) -> N/1

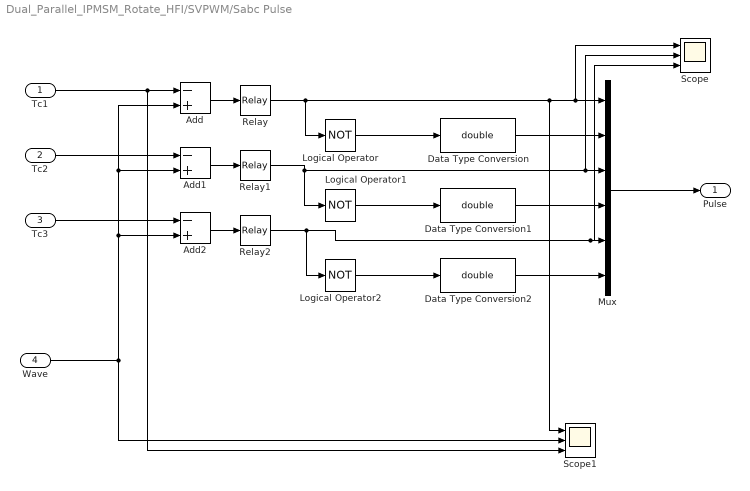
== system Dual_Parallel_IPMSM_Rotate_HFI/SVPWM/Sabc Pulse ==
  Tc1 : Inport
  Tc2 : Inport  Port=2
  Tc3 : Inport  Port=3
  Wave : Inport  Port=4
  Add : Sum  Inputs=-+
  Add1 : Sum  Inputs=-+
  Add2 : Sum  Inputs=-+
  Data Type Conversion : DataTypeConversion  OutDataTypeStr=double  SaturateOnIntegerOverflow=off  RndMeth=Floor
  Data Type Conversion1 : DataTypeConversion  OutDataTypeStr=double  SaturateOnIntegerOverflow=off  RndMeth=Floor
  Data Type Conversion2 : DataTypeConversion  OutDataTypeStr=double  SaturateOnIntegerOverflow=off  RndMeth=Floor
  Logical Operator : Logic  Operator=NOT  AllPortsSameDT=off  OutDataTypeStr=boolean
  Logical Operator1 : Logic  Operator=NOT  AllPortsSameDT=off  OutDataTypeStr=boolean
  Logical Operator2 : Logic  Operator=NOT  AllPortsSameDT=off  OutDataTypeStr=boolean
  Mux : Mux  Inputs=6
  Relay : Relay
  Relay1 : Relay
  Relay2 : Relay
  Scope : Scope  NumInputPorts=3
  Scope1 : Scope  NumInputPorts=3
  "Pulse " : Outport  VectorParamsAs1DForOutWhenUnconnected=off
  wires:
  Add/1 -> Relay/1
  Add1/1 -> Relay1/1
  Wave/1 -> Add2/2, Add1/2, Add/2, Scope1/2
  Tc2/1 -> Add1/1
  Tc1/1 -> Scope1/3, Add/1
  Tc3/1 -> Add2/1
  Logical Operator/1 -> Data Type Conversion/1
  Logical Operator1/1 -> Data Type Conversion1/1
  Add2/1 -> Relay2/1
  Logical Operator2/1 -> Data Type Conversion2/1
  Mux/1 -> "Pulse "/1
  Relay/1 -> Scope1/1, Scope/1, Mux/1, Logical Operator/1
  Relay1/1 -> Scope/2, Mux/3, Logical Operator1/1
  Relay2/1 -> Logical Operator2/1, Scope/3, Mux/5
  Data Type Conversion/1 -> Mux/2
  Data Type Conversion1/1 -> Mux/4
  Data Type Conversion2/1 -> Mux/6

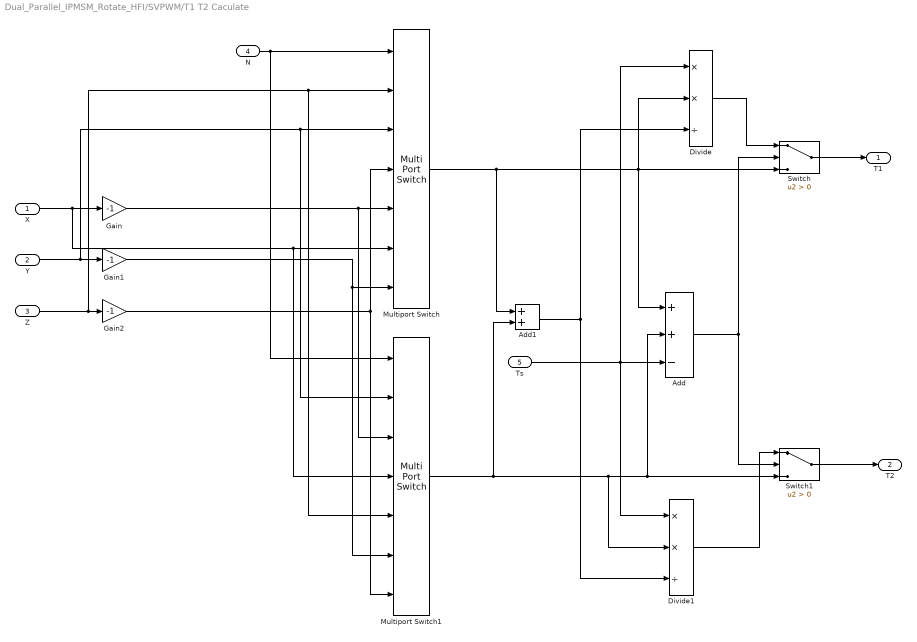
== system Dual_Parallel_IPMSM_Rotate_HFI/SVPWM/T1 T2 Caculate ==
  X : Inport
  Y : Inport  Port=2
  Z : Inport  Port=3
  N : Inport  Port=4
  "Ts " : Inport  Port=5
  Add : Sum  Inputs=++-
  Add1 : Sum
  Divide : Product  Inputs=**/
  Divide1 : Product  Inputs=**/
  Gain : Gain  Gain=-1
  Gain1 : Gain  Gain=-1
  Gain2 : Gain  Gain=-1
  Multiport Switch : MultiPortSwitch  Inputs=6  SaturateOnIntegerOverflow=off  InputSameDT=off
  Multiport Switch1 : MultiPortSwitch  Inputs=6  SaturateOnIntegerOverflow=off  InputSameDT=off
  Switch : Switch  Criteria=u2 > Threshold  SaturateOnIntegerOverflow=off  InputSameDT=off
  Switch1 : Switch  Criteria=u2 > Threshold  SaturateOnIntegerOverflow=off  InputSameDT=off
  T1 : Outport  VectorParamsAs1DForOutWhenUnconnected=off
  T2 : Outport  Port=2  VectorParamsAs1DForOutWhenUnconnected=off
  wires:
  Y/1 -> Multiport Switch1/2, Multiport Switch/3, Gain1/1
  X/1 -> Multiport Switch1/4, Multiport Switch/6, Gain/1
  N/1 -> Multiport Switch/1, Multiport Switch1/1
  Z/1 -> Multiport Switch1/5, Multiport Switch/2, Gain2/1
  Gain2/1 -> Multiport Switch1/7, Multiport Switch/4
  Gain/1 -> Multiport Switch1/3, Multiport Switch/5
  Gain1/1 -> Multiport Switch1/6, Multiport Switch/7
  Multiport Switch/1 -> Add1/1, Divide/2, Add/1, Switch/3
  Multiport Switch1/1 -> Add1/2, Divide1/2, Add/2, Switch1/3
  "Ts "/1 -> Divide1/1, Divide/1, Add/3
  Add/1 -> Switch1/2, Switch/2
  Divide/1 -> Switch/1
  Add1/1 -> Divide/3, Divide1/3
  Switch/1 -> T1/1
  Switch1/1 -> T2/1
  Divide1/1 -> Switch1/1

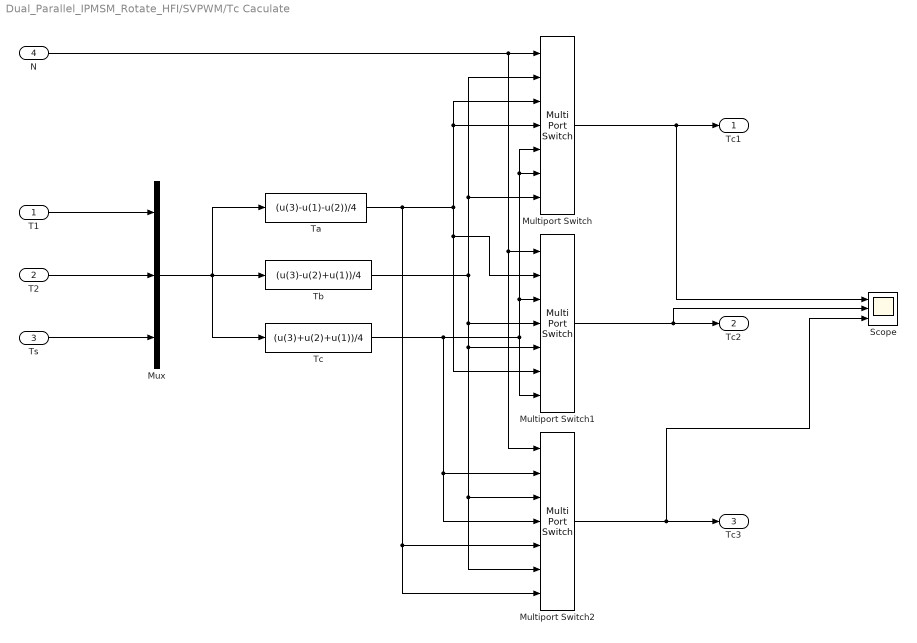
== system Dual_Parallel_IPMSM_Rotate_HFI/SVPWM/Tc Caculate ==
  T1 : Inport
  T2 : Inport  Port=2
  Ts : Inport  Port=3
  N : Inport  Port=4
  Multiport Switch : MultiPortSwitch  Inputs=6  SaturateOnIntegerOverflow=off  InputSameDT=off
  Multiport Switch1 : MultiPortSwitch  Inputs=6  SaturateOnIntegerOverflow=off  InputSameDT=off
  Multiport Switch2 : MultiPortSwitch  Inputs=6  SaturateOnIntegerOverflow=off  InputSameDT=off
  Mux : Mux  Inputs=3
  Scope : Scope  NumInputPorts=3
  Ta : Fcn  Expr=(u(3)-u(1)-u(2))/4
  Tb : Fcn  Expr=(u(3)-u(2)+u(1))/4
  Tc : Fcn  Expr=(u(3)+u(2)+u(1))/4
  Tc1 : Outport  VectorParamsAs1DForOutWhenUnconnected=off
  Tc2 : Outport  Port=2  VectorParamsAs1DForOutWhenUnconnected=off
  Tc3 : Outport  Port=3  VectorParamsAs1DForOutWhenUnconnected=off
  wires:
  T2/1 -> Mux/2
  T1/1 -> Mux/1
  Ts/1 -> Mux/3
  Mux/1 -> Tc/1, Ta/1, Tb/1
  N/1 -> Multiport Switch2/1, Multiport Switch1/1, Multiport Switch/1
  Ta/1 -> Multiport Switch2/7, Multiport Switch2/5, Multiport Switch/3, Multiport Switch/4, Multiport Switch1/6, Multiport Switch1/2
  Tb/1 -> Multiport Switch/7, Multiport Switch/2, Multiport Switch1/4, Multiport Switch2/6, Multiport Switch2/3, Multiport Switch1/5
  Tc/1 -> Multiport Switch2/4, Multiport Switch2/2, Multiport Switch1/7, Multiport Switch1/3, Multiport Switch/6, Multiport Switch/5
  Multiport Switch/1 -> Scope/1, Tc1/1
  Multiport Switch1/1 -> Scope/2, Tc2/1
  Multiport Switch2/1 -> Scope/3, Tc3/1

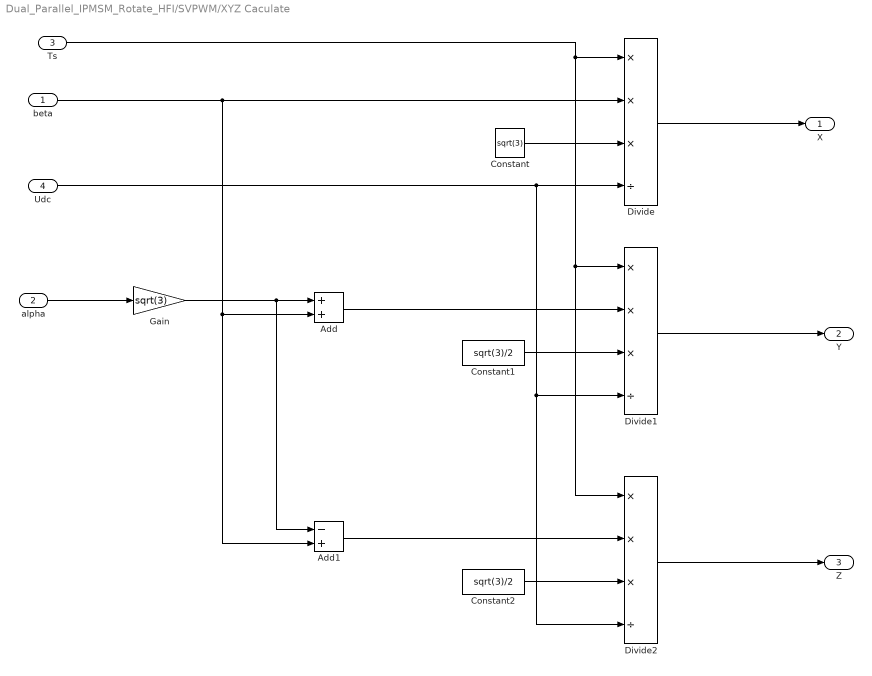
== system Dual_Parallel_IPMSM_Rotate_HFI/SVPWM/XYZ Caculate ==
  beta : Inport
  alpha : Inport  Port=2
  "Ts " : Inport  Port=3
  Udc : Inport  Port=4
  Add : Sum
  Add1 : Sum  Inputs=-+
  Constant : Constant  Value=sqrt(3)
  Constant1 : Constant  Value=sqrt(3)/2
  Constant2 : Constant  Value=sqrt(3)/2
  Divide : Product  Inputs=***/
  Divide1 : Product  Inputs=***/
  Divide2 : Product  Inputs=***/
  Gain : Gain  Gain=sqrt(3)
  X : Outport  VectorParamsAs1DForOutWhenUnconnected=off
  Y : Outport  Port=2  VectorParamsAs1DForOutWhenUnconnected=off
  Z : Outport  Port=3  VectorParamsAs1DForOutWhenUnconnected=off
  wires:
  "Ts "/1 -> Divide2/1, Divide1/1, Divide/1
  Udc/1 -> Divide1/4, Divide2/4, Divide/4
  Constant/1 -> Divide/3
  beta/1 -> Add1/2, Add/2, Divide/2
  Constant2/1 -> Divide2/3
  Constant1/1 -> Divide1/3
  Add/1 -> Divide1/2
  Add1/1 -> Divide2/2
  Gain/1 -> Add1/1, Add/1
  alpha/1 -> Gain/1
  Divide1/1 -> Y/1
  Divide/1 -> X/1
  Divide2/1 -> Z/1

== matlab function Dual_Parallel_IPMSM_Rotate_HFI/MATLAB Function1 ==
  data: alpha input; d output; beta input; theta_e input; q output
function [d,q] = alphabeta_to_dq(alpha,beta,theta_e)

d = cos(theta_e) * alpha + sin(theta_e) * beta;
q = - sin(theta_e) * alpha + cos(theta_e) * beta;

== matlab function Dual_Parallel_IPMSM_Rotate_HFI/MATLAB Function ==
  data: a input; alpha output; b input; c input; beta output
function [alpha,beta] = abc_to_alphabeta(a,b,c)

alpha = (2/3) * (a - 0.5 * b - 0.5 * c);
beta = sqrt(3)/3 * (b-c);

== matlab function Dual_Parallel_IPMSM_Rotate_HFI/Speed_calc/MATLAB Function2 ==
  data: theta_m2 input; theta_m1 input; speed_m output; speed_m1 input; speed_init input; fc input; t input
function speed_m = speed_calc(theta_m2, theta_m1, speed_m1, speed_init, fc, t)

speed_m2 = (theta_m2 - theta_m1)/(1e-4);

low_pass_factor1 = 2 * pi * fc * 1e-4;
low_pass_factor2 = low_pass_factor1 / (1 + low_pass_factor1);

speed_m = low_pass_factor2 * speed_m2 + (1 - low_pass_factor2) * speed_m1;

if t == 0
    speed_m = speed_init;
end

end

== matlab function Dual_Parallel_IPMSM_Rotate_HFI/MATLAB Function2 ==
  data: d input; alpha output; q input; theta_e input; beta output
function [alpha,beta] = dq_to_alphabeta(d, q, theta_e)

alpha = d * cos(theta_e) - q * sin(theta_e);
beta = d * sin(theta_e) + q * cos(theta_e);

== matlab function Dual_Parallel_IPMSM_Rotate_HFI/SVPWM/N Caculate/MATLAB Function ==
  data: u input; y output
function y = fcn(u)
if u==0
    y=1;
else
    y = u;
end

== matlab function Dual_Parallel_IPMSM_Rotate_HFI/Theta_scope1/MATLAB Function ==
  data: theta input; theta_normalize output
function theta_normalize = fcn(theta)
if (theta > pi)
    theta = theta - 2 * pi;
elseif (theta< -pi)
    theta = theta + 2 * pi;
end
theta_normalize = theta;

== matlab function Dual_Parallel_IPMSM_Rotate_HFI/Theta_scope1/MATLAB Function1 ==
  data: theta input; theta_normalize output
function theta_normalize = fcn(theta)
if (theta > pi)
    theta = theta - 2 * pi;
elseif (theta< -pi)
    theta = theta + 2 * pi;
end
theta_normalize = theta;

== matlab function Dual_Parallel_IPMSM_Rotate_HFI/Theta_scope1/MATLAB Function2 ==
  data: theta input; theta_normalize output
function theta_normalize = fcn(theta)
if (theta > pi)
    theta = theta - 2 * pi;
elseif (theta< -pi)
    theta = theta + 2 * pi;
end
theta_normalize = theta;

== matlab function Dual_Parallel_IPMSM_Rotate_HFI/MATLAB Function3 ==
  data: ec input; theta_d output; es input
function theta_d = theta_d_calc(ec, es)

    eps = 1e-4;
    if abs(ec) < eps
        if abs(es) < eps
            theta_d = 0;
        else
            theta_d = pi/2;
        end
    else
        theta_d = atan(-es / ec);
    end

end
